simulink model "CM670A_HwAg1Meas"  (R2013b)
settings: Solver=FixedStepDiscrete  SolverMode=SingleTasking  StartTime=0.0  StopTime=22  FixedStep=0.002  RelTol=1e-3
values from neighbouring files (symbols this model uses):
  ELECGLBPRM_DEGPERREV_DEGPERREV_F32 = DataDict.Constant    [CM670A_HwAg1Meas_DataDict.m]
  ELECGLBPRM_HWAGCENTROFFS_HWDEG_F32 = DataDict.Constant    [CM670A_HwAg1Meas_DataDict.m]
  ELECGLBPRM_HWAGSATNLOWRLIM_HWDEG_F32 = DataDict.Constant    [CM670A_HwAg1Meas_DataDict.m]
  ELECGLBPRM_HWAGSATNUPPRLIM_HWDEG_F32 = DataDict.Constant    [CM670A_HwAg1Meas_DataDict.m]
  ELECGLBPRM_HWAGSCA_ULS_F32 = DataDict.Constant    [CM670A_HwAg1Meas_DataDict.m]
  ELECGLBPRM_HWAGSPURGEARRAT_ULS_F32 = DataDict.Constant    [CM670A_HwAg1Meas_DataDict.m]
  ELECGLBPRM_HWAGSPURTORINGGEARRATSNSR0_ULS_F32 = DataDict.Constant    [CM670A_HwAg1Meas_DataDict.m]
  ELECGLBPRM_HWAGSPURTORINGGEARRATSNSR1_ULS_F32 = DataDict.Constant    [CM670A_HwAg1Meas_DataDict.m]
  ELECGLBPRM_NOFLT_CNT_U08 = DataDict.Constant    [CM670A_HwAg1Meas_DataDict.m]
  ELECGLBPRM_OFFSTRIMNOTPRFMD_CNT_U08 = DataDict.Constant    [CM670A_HwAg1Meas_DataDict.m]
  ELECGLBPRM_PRTCLFLT_CNT_U08 = DataDict.Constant    [CM670A_HwAg1Meas_DataDict.m]
  ELECGLBPRM_SKIPSTEPFLT_CNT_U08 = DataDict.Constant    [CM670A_HwAg1Meas_DataDict.m]
  ELECGLBPRM_SNSRINTFLT_CNT_U08 = DataDict.Constant    [CM670A_HwAg1Meas_DataDict.m]
  ELECGLBPRM_VRNRERRFLT_CNT_U08 = DataDict.Constant    [CM670A_HwAg1Meas_DataDict.m]
  HWAG10THTOOTHTRIG_CNT_U08 = DataDict.ConfigParam    [CM670A_HwAg1Meas_DataDict.m]
  HWAG11THTOOTHTRIG_CNT_U08 = DataDict.ConfigParam    [CM670A_HwAg1Meas_DataDict.m]
  HwAg1IfFlt = DataDict.NTC    [CM670A_HwAg1Meas_DataDict.m]
  HwAg1MeasHwAg1IfFltFailStep = DataDict.Calibration    [CM670A_HwAg1Meas_DataDict.m]
  HwAg1MeasHwAg1IfFltPassStep = DataDict.Calibration    [CM670A_HwAg1Meas_DataDict.m]
  HwAg1MeasHwAg1Snsr0PrtclFltFailStep = DataDict.Calibration    [CM670A_HwAg1Meas_DataDict.m]
  HwAg1MeasHwAg1Snsr0PrtclFltPassStep = DataDict.Calibration    [CM670A_HwAg1Meas_DataDict.m]
  HwAg1MeasHwAg1Snsr1PrtclFltFailStep = DataDict.Calibration    [CM670A_HwAg1Meas_DataDict.m]
  HwAg1MeasHwAg1Snsr1PrtclFltPassStep = DataDict.Calibration    [CM670A_HwAg1Meas_DataDict.m]
  HwAg1MeasSnsr0Rev = DataDict.Calibration    [CM670A_HwAg1Meas_DataDict.m]
  HwAg1MeasSnsr1Rev = DataDict.Calibration    [CM670A_HwAg1Meas_DataDict.m]
  HwAg1MeasStep = DataDict.Calibration    [CM670A_HwAg1Meas_DataDict.m]
  HwAg1MeasVrnrErrThd = DataDict.Calibration    [CM670A_HwAg1Meas_DataDict.m]
  HwAg1MfgFlt = DataDict.NTC    [CM670A_HwAg1Meas_DataDict.m]
  HwAg1Snsr0PrtclFlt = DataDict.NTC    [CM670A_HwAg1Meas_DataDict.m]
  HwAg1Snsr1PrtclFlt = DataDict.NTC    [CM670A_HwAg1Meas_DataDict.m]
undefined symbols (not defined in the file or in its folder): NtcSts1, sigbuilder_block, SigQlfr1
libraries: simulink x30, NxtrNvM x3
(part 5 of 5)

== system CM670A_HwAg1Meas/HwAg1Meas/HwAg1MeasPer2/Snsr0Read/RawHwAgRead/NewMsg/NoStsFlt/CommFlt ==
  Action Port : ActionPort  ActionType=else
  Add : Sum
  Bus Creator1 : BusCreator  Inputs=3
  Constant : Constant  OutDataTypeStr=uint8
  CopyRight2 : Subsystem  Description=|  mask(Copyright Information){none=on}
      | Copyright info block.                                               
      |                                                                     
      | Place copyright information at the top of every subsystem in design.
      mask prompts: none "No parameters"
      mask help: Place copyright information at the top of every subsystem in design.
      mask Display:
      | NxtrConf = 'Nexteer Confidential';
      | 
      | sys = bdroot; %handle for the current model ("system")
      | first = get_param(sys,'Created');
      | first = first(end-3:end);  %year is last four digits
      | 
      | last = get_param(sys,'LastModifiedDate');
      | if isempty(last)
      |     last = datestr(now,'yyyy');
      | else
      |     last = last(end-3:end);
      | end
      | 
      | if strcmp(first,last)
      |     fprintf('%s -- Copyright %s Nexteer',NxtrConf,first)
      | else
      |     fprintf('%s -- %s%s- %s Nexteer',NxtrConf,char(169),first,last)
      | end
  Data Store Read : DataStoreRead  DataStoreName=HwAg1Snsr0IntSnsrErrCntr
  Data Store Write : DataStoreWrite  DataStoreName=HwAg1Snsr0IntSnsrErrCntr
  Data Type Conversion : DataTypeConversion  OutDataTypeStr=uint8
  Flt : Constant  Value=ELECGLBPRM_SNSRINTFLT_CNT_U08  OutDataTypeStr=uint8
  HwAg : Constant  Value=0  OutDataTypeStr=uint16
  NtcSts : simulink/Sources/Enumerated Constant  OutDataTypeStr=Enum: NtcSts1  Value=NtcSts1.NTCSTS_PREFAILD  SampleTime=inf
  Signal Conversion1 : SignalConversion
  Out2 : Outport
  wires:
  Flt/1 -> Bus Creator1/3  "ParamByte"
  NtcSts/1 -> Data Type Conversion/1
  HwAg/1 -> Bus Creator1/1  "RawHwAg"
  Bus Creator1/1 -> Signal Conversion1/1
  Signal Conversion1/1 -> Out2/1
  Data Type Conversion/1 -> Bus Creator1/2  "TestOk"
  Data Store Read/1 -> Add/1
  Constant/1 -> Add/2
  Add/1 -> Data Store Write/1

== system CM670A_HwAg1Meas/HwAg1Meas/HwAg1MeasPer2/Snsr0Read/RawHwAgRead/NewMsg/NoStsFlt/CopyRight2 ==

== system CM670A_HwAg1Meas/HwAg1Meas/HwAg1MeasPer2/Snsr0Read/RawHwAgRead/NewMsg/NoStsFlt/TestPass ==
  Snsr0Id : Inport
  Snsr0Data : Inport  Port=2
  Action Port : ActionPort  ActionType=then
  Bus Creator : BusCreator  Inputs=3
  CopyRight2 : Subsystem  Description=|  mask(Copyright Information){none=on}
      | Copyright info block.                                               
      |                                                                     
      | Place copyright information at the top of every subsystem in design.
      mask prompts: none "No parameters"
      mask help: Place copyright information at the top of every subsystem in design.
      mask Display:
      | NxtrConf = 'Nexteer Confidential';
      | 
      | sys = bdroot; %handle for the current model ("system")
      | first = get_param(sys,'Created');
      | first = first(end-3:end);  %year is last four digits
      | 
      | last = get_param(sys,'LastModifiedDate');
      | if isempty(last)
      |     last = datestr(now,'yyyy');
      | else
      |     last = last(end-3:end);
      | end
      | 
      | if strcmp(first,last)
      |     fprintf('%s -- Copyright %s Nexteer',NxtrConf,first)
      | else
      |     fprintf('%s -- %s%s- %s Nexteer',NxtrConf,char(169),first,last)
      | end
  If Action Subsystem : Subsystem  RequirementInfo={'linktype_rmi_doors' '0000cf44 (/ESG Group/FDD Module Requirements/EA4 Specific/CM670A_HwAg1Meas)' '#CM670A_49' 'true' 'REQ: CM670A_49' '' } %GIDa_aa48b249_ab70_46ce_8963_12185f434e4c  TreatAsAtomicUnit=on
  If Action Subsystem2 : Subsystem  RequirementInfo={'linktype_rmi_doors' '0000cf44 (/ESG Group/FDD Module Requirements/EA4 Specific/CM670A_HwAg1Meas)' '#CM670A_74' 'true' 'REQ: CM670A_74' '' } %GIDa_f5c78345_3720_4b83_a791_e0c886f64c70  TreatAsAtomicUnit=on
  If2 : If  IfExpression=u1 == 0
  Merge : Merge
  Merge1 : Merge
  Merge2 : Merge
  Out1 : Outport
  wires:
  Merge1/1 -> Bus Creator/2  "TestOk"
  Merge2/1 -> Bus Creator/3  "ParamByte"
  Merge/1 -> Bus Creator/1  "RawHwAg"
  Bus Creator/1 -> Out1/1
  Snsr0Id/1 -> If2/1
  If2/1 -> If Action Subsystem/Action
  If2/2 -> If Action Subsystem2/Action
  If Action Subsystem/1(RawHwAg) -> Merge/1
  If Action Subsystem2/1(RawHwAg) -> Merge/2
  If Action Subsystem/2(NtcSts) -> Merge1/1
  If Action Subsystem2/2(NtcSts) -> Merge1/2
  If Action Subsystem/3(ParamByte) -> Merge2/1
  If Action Subsystem2/3(ParamByte) -> Merge2/2
  Snsr0Data/1 -> If Action Subsystem/1(Snsr0Data)

== system CM670A_HwAg1Meas/HwAg1Meas/HwAg1MeasPer2/Snsr0Read/RawHwAgRead/NewMsg/STSFLT/CopyRight2 ==

== system CM670A_HwAg1Meas/HwAg1Meas/HwAg1MeasPer3/Snsr1Read/RawHwAgRead/NewMsg/NoStsFlt/CommFlt ==
  Action Port : ActionPort  ActionType=else
  Add : Sum
  Bus Creator1 : BusCreator  Inputs=3
  Constant : Constant  OutDataTypeStr=uint8
  CopyRight2 : Subsystem  Description=|  mask(Copyright Information){none=on}
      | Copyright info block.                                               
      |                                                                     
      | Place copyright information at the top of every subsystem in design.
      mask prompts: none "No parameters"
      mask help: Place copyright information at the top of every subsystem in design.
      mask Display:
      | NxtrConf = 'Nexteer Confidential';
      | 
      | sys = bdroot; %handle for the current model ("system")
      | first = get_param(sys,'Created');
      | first = first(end-3:end);  %year is last four digits
      | 
      | last = get_param(sys,'LastModifiedDate');
      | if isempty(last)
      |     last = datestr(now,'yyyy');
      | else
      |     last = last(end-3:end);
      | end
      | 
      | if strcmp(first,last)
      |     fprintf('%s -- Copyright %s Nexteer',NxtrConf,first)
      | else
      |     fprintf('%s -- %s%s- %s Nexteer',NxtrConf,char(169),first,last)
      | end
  Data Store Read : DataStoreRead  DataStoreName=HwAg1Snsr1IntSnsrErrCntr
  Data Store Write : DataStoreWrite  DataStoreName=HwAg1Snsr1IntSnsrErrCntr
  Data Type Conversion : DataTypeConversion  OutDataTypeStr=uint8
  Flt : Constant  Value=ELECGLBPRM_SNSRINTFLT_CNT_U08  OutDataTypeStr=uint8
  HwAg : Constant  Value=0  OutDataTypeStr=uint16
  NtcSts : simulink/Sources/Enumerated Constant  OutDataTypeStr=Enum: NtcSts1  Value=NtcSts1.NTCSTS_PREFAILD  SampleTime=inf
  Signal Conversion1 : SignalConversion
  Out2 : Outport
  wires:
  Flt/1 -> Bus Creator1/3  "ParamByte"
  NtcSts/1 -> Data Type Conversion/1
  HwAg/1 -> Bus Creator1/1  "RawHwAg"
  Bus Creator1/1 -> Signal Conversion1/1
  Signal Conversion1/1 -> Out2/1
  Data Type Conversion/1 -> Bus Creator1/2  "TestOk"
  Data Store Read/1 -> Add/1
  Constant/1 -> Add/2
  Add/1 -> Data Store Write/1

== system CM670A_HwAg1Meas/HwAg1Meas/HwAg1MeasPer3/Snsr1Read/RawHwAgRead/NewMsg/NoStsFlt/CopyRight2 ==

== system CM670A_HwAg1Meas/HwAg1Meas/HwAg1MeasPer3/Snsr1Read/RawHwAgRead/NewMsg/NoStsFlt/TestPass ==
  Snsr1Id : Inport
  Snsr1Data : Inport  Port=2
  Action Port : ActionPort  ActionType=then
  Bus Creator : BusCreator  Inputs=3
  CopyRight2 : Subsystem  Description=|  mask(Copyright Information){none=on}
      | Copyright info block.                                               
      |                                                                     
      | Place copyright information at the top of every subsystem in design.
      mask prompts: none "No parameters"
      mask help: Place copyright information at the top of every subsystem in design.
      mask Display:
      | NxtrConf = 'Nexteer Confidential';
      | 
      | sys = bdroot; %handle for the current model ("system")
      | first = get_param(sys,'Created');
      | first = first(end-3:end);  %year is last four digits
      | 
      | last = get_param(sys,'LastModifiedDate');
      | if isempty(last)
      |     last = datestr(now,'yyyy');
      | else
      |     last = last(end-3:end);
      | end
      | 
      | if strcmp(first,last)
      |     fprintf('%s -- Copyright %s Nexteer',NxtrConf,first)
      | else
      |     fprintf('%s -- %s%s- %s Nexteer',NxtrConf,char(169),first,last)
      | end
  If Action Subsystem : Subsystem  RequirementInfo={'linktype_rmi_doors' '0000cf44 (/ESG Group/FDD Module Requirements/EA4 Specific/CM670A_HwAg1Meas)' '#CM670A_73' 'true' 'REQ: CM670A_73' '' } %GIDa_606bd5a3_5e49_4a65_919f_9ded041dacb2  TreatAsAtomicUnit=on
  If Action Subsystem2 : Subsystem  RequirementInfo={'linktype_rmi_doors' '0000cf44 (/ESG Group/FDD Module Requirements/EA4 Specific/CM670A_HwAg1Meas)' '#CM670A_75' 'true' 'REQ: CM670A_75' '' } %GIDa_005b1b66_d003_4573_abd6_345df925bde0  TreatAsAtomicUnit=on
  If2 : If  IfExpression=u1 == 1
  Merge : Merge
  Merge1 : Merge
  Merge2 : Merge
  Out1 : Outport
  wires:
  Merge1/1 -> Bus Creator/2  "TestOk"
  Merge2/1 -> Bus Creator/3  "ParamByte"
  Merge/1 -> Bus Creator/1  "RawHwAg"
  Bus Creator/1 -> Out1/1
  Snsr1Id/1 -> If2/1
  If2/1 -> If Action Subsystem/Action
  If2/2 -> If Action Subsystem2/Action
  If Action Subsystem/1(RawHwAg) -> Merge/1
  If Action Subsystem2/1(RawHwAg) -> Merge/2
  If Action Subsystem/2(NtcSts) -> Merge1/1
  If Action Subsystem2/2(NtcSts) -> Merge1/2
  If Action Subsystem/3(ParamByte) -> Merge2/1
  If Action Subsystem2/3(ParamByte) -> Merge2/2
  Snsr1Data/1 -> If Action Subsystem/1(Snsr1Data)

== system CM670A_HwAg1Meas/HwAg1Meas/HwAg1MeasPer3/Snsr1Read/RawHwAgRead/NewMsg/STSFLT/CopyRight2 ==

== system CM670A_HwAg1Meas/HwAg1Meas/HwAg1MeasPer4/HwAgRead/If Action Subsystem/AdjStepCalc/Diagc/CopyRight2 ==

== system CM670A_HwAg1Meas/HwAg1Meas/HwAg1MeasPer4/HwAgRead/If Action Subsystem/AdjStepCalc/Diagc/If Action  ==
  HwAg1Snsr0Rev : Inport
  HwAg1Snsr1Rev : Inport  Port=2
  HwAg1Snsr0Rel : Inport  Port=3
  HwAg1Snsr1Rel : Inport  Port=4
  HwAg1StepSeqNr : Inport  Port=5
  Action Port : ActionPort  ActionType=then
  AbsCalcHwAg1Snsr0 : Subsystem
  AbsCalcHwAg1Snsr1 : Subsystem
  CopyRight2 : Subsystem  Description=|  mask(Copyright Information){none=on}
      | Copyright info block.                                               
      |                                                                     
      | Place copyright information at the top of every subsystem in design.
      mask prompts: none "No parameters"
      mask help: Place copyright information at the top of every subsystem in design.
      mask Display:
      | NxtrConf = 'Nexteer Confidential';
      | 
      | sys = bdroot; %handle for the current model ("system")
      | first = get_param(sys,'Created');
      | first = first(end-3:end);  %year is last four digits
      | 
      | last = get_param(sys,'LastModifiedDate');
      | if isempty(last)
      |     last = datestr(now,'yyyy');
      | else
      |     last = last(end-3:end);
      | end
      | 
      | if strcmp(first,last)
      |     fprintf('%s -- Copyright %s Nexteer',NxtrConf,first)
      | else
      |     fprintf('%s -- %s%s- %s Nexteer',NxtrConf,char(169),first,last)
      | end
  PIM : DataStoreWrite  DataStoreName=HwAg1PrevStepSeqNr
  finalAbsAg : Subsystem
  HwAg1Meas : Outport
  HwAg1TestOk : Outport  Port=2
  ParamByte : Outport  Port=3
  wires:
  HwAg1Snsr0Rev/1 -> AbsCalcHwAg1Snsr0/2(HwAg1Snsr0Rev)
  AbsCalcHwAg1Snsr0/1(HwAg1Snsr0Abs) -> finalAbsAg/1(HwAg1Snsr0Abs)
  AbsCalcHwAg1Snsr1/1(HwAg1Snsr1Abs) -> finalAbsAg/2(HwAg1Snsr1Abs)
  finalAbsAg/1(HwAg1) -> HwAg1Meas/1
  finalAbsAg/2(TestOk) -> HwAg1TestOk/1
  finalAbsAg/3(ParamByte) -> ParamByte/1
  HwAg1Snsr0Rel/1 -> AbsCalcHwAg1Snsr0/1(HwAg1Snsr0Rel)
  HwAg1StepSeqNr/1 -> PIM/1
  HwAg1Snsr1Rel/1 -> AbsCalcHwAg1Snsr1/1(HwAg1Snsr1Rel)
  HwAg1Snsr1Rev/1 -> AbsCalcHwAg1Snsr1/2(HwAg1Snsr1Rev)

== system CM670A_HwAg1Meas/HwAg1Meas/HwAg1MeasPer4/HwAgRead/If Action Subsystem/AdjStepCalc/Diagc/If Action Skip ==
  Action Port : ActionPort  ActionType=else
  CopyRight2 : Subsystem  Description=|  mask(Copyright Information){none=on}
      | Copyright info block.                                               
      |                                                                     
      | Place copyright information at the top of every subsystem in design.
      mask prompts: none "No parameters"
      mask help: Place copyright information at the top of every subsystem in design.
      mask Display:
      | NxtrConf = 'Nexteer Confidential';
      | 
      | sys = bdroot; %handle for the current model ("system")
      | first = get_param(sys,'Created');
      | first = first(end-3:end);  %year is last four digits
      | 
      | last = get_param(sys,'LastModifiedDate');
      | if isempty(last)
      |     last = datestr(now,'yyyy');
      | else
      |     last = last(end-3:end);
      | end
      | 
      | if strcmp(first,last)
      |     fprintf('%s -- Copyright %s Nexteer',NxtrConf,first)
      | else
      |     fprintf('%s -- %s%s- %s Nexteer',NxtrConf,char(169),first,last)
      | end
  Data Type Conversion : DataTypeConversion  OutDataTypeStr=uint8
  Flt : Constant  Value=ELECGLBPRM_SKIPSTEPFLT_CNT_U08  OutDataTypeStr=uint8
  HwAg1 : Constant  Value=0  OutDataTypeStr=single
  NtcSts : simulink/Sources/Enumerated Constant  OutDataTypeStr=Enum: NtcSts1  Value=NtcSts1.NTCSTS_PREFAILD  SampleTime=inf
  HwAg1Meas : Outport
  HwAg1TestOk : Outport  Port=2  OutDataTypeStr=uint8
  ParamByte : Outport  Port=3
  wires:
  NtcSts/1 -> Data Type Conversion/1
  Flt/1 -> ParamByte/1
  HwAg1/1 -> HwAg1Meas/1
  Data Type Conversion/1 -> HwAg1TestOk/1

== system CM670A_HwAg1Meas/HwAg1Meas/HwAg1MeasPer4/HwAgRead/If Action Subsystem/AdjStepCalc/InitStep/CopyRight2 ==

== system CM670A_HwAg1Meas/HwAg1Meas/HwAg1MeasPer4/HwAgRead/If Action Subsystem/AdjStepCalc/InitStep/DoNothing ==
  Action Port : ActionPort  ActionType=else
  CopyRight2 : Subsystem  Description=|  mask(Copyright Information){none=on}
      | Copyright info block.                                               
      |                                                                     
      | Place copyright information at the top of every subsystem in design.
      mask prompts: none "No parameters"
      mask help: Place copyright information at the top of every subsystem in design.
      mask Display:
      | NxtrConf = 'Nexteer Confidential';
      | 
      | sys = bdroot; %handle for the current model ("system")
      | first = get_param(sys,'Created');
      | first = first(end-3:end);  %year is last four digits
      | 
      | last = get_param(sys,'LastModifiedDate');
      | if isempty(last)
      |     last = datestr(now,'yyyy');
      | else
      |     last = last(end-3:end);
      | end
      | 
      | if strcmp(first,last)
      |     fprintf('%s -- Copyright %s Nexteer',NxtrConf,first)
      | else
      |     fprintf('%s -- %s%s- %s Nexteer',NxtrConf,char(169),first,last)
      | end

== system CM670A_HwAg1Meas/HwAg1Meas/HwAg1MeasPer4/HwAgRead/If Action Subsystem/AdjStepCalc/InitStep/Else ==
  HwAg1StepSeqNr : Inport
  Action Port : ActionPort  ActionType=then
  Constant : Constant  OutDataTypeStr=boolean
  CopyRight2 : Subsystem  Description=|  mask(Copyright Information){none=on}
      | Copyright info block.                                               
      |                                                                     
      | Place copyright information at the top of every subsystem in design.
      mask prompts: none "No parameters"
      mask help: Place copyright information at the top of every subsystem in design.
      mask Display:
      | NxtrConf = 'Nexteer Confidential';
      | 
      | sys = bdroot; %handle for the current model ("system")
      | first = get_param(sys,'Created');
      | first = first(end-3:end);  %year is last four digits
      | 
      | last = get_param(sys,'LastModifiedDate');
      | if isempty(last)
      |     last = datestr(now,'yyyy');
      | else
      |     last = last(end-3:end);
      | end
      | 
      | if strcmp(first,last)
      |     fprintf('%s -- Copyright %s Nexteer',NxtrConf,first)
      | else
      |     fprintf('%s -- %s%s- %s Nexteer',NxtrConf,char(169),first,last)
      | end
  PIM : DataStoreWrite  DataStoreName=HwAg1PrevStepSeqNr
  PIM1 : DataStoreWrite  DataStoreName=HwAg1InitStepSeqNrCmpl
  wires:
  HwAg1StepSeqNr/1 -> PIM/1
  Constant/1 -> PIM1/1

== system CM670A_HwAg1Meas/HwAg1Meas/HwAg1MeasPer4/HwAgRead/If Action Subsystem/AdjStepCalc/Intpn/CopyRight2 ==

== system CM670A_HwAg1Meas/HwAg1Meas/HwAg1MeasPer4/HwAgRead/If Action Subsystem/AdjStepCalc/Intpn/StepCalc ==
  HwAg1Snsr0Rel : Inport
  HwAg1Snsr1Rel : Inport  Port=2
  Add : Sum  Inputs=+-
  CopyRight2 : Subsystem  Description=|  mask(Copyright Information){none=on}
      | Copyright info block.                                               
      |                                                                     
      | Place copyright information at the top of every subsystem in design.
      mask prompts: none "No parameters"
      mask help: Place copyright information at the top of every subsystem in design.
      mask Display:
      | NxtrConf = 'Nexteer Confidential';
      | 
      | sys = bdroot; %handle for the current model ("system")
      | first = get_param(sys,'Created');
      | first = first(end-3:end);  %year is last four digits
      | 
      | last = get_param(sys,'LastModifiedDate');
      | if isempty(last)
      |     last = datestr(now,'yyyy');
      | else
      |     last = last(end-3:end);
      | end
      | 
      | if strcmp(first,last)
      |     fprintf('%s -- Copyright %s Nexteer',NxtrConf,first)
      | else
      |     fprintf('%s -- %s%s- %s Nexteer',NxtrConf,char(169),first,last)
      | end
  Data Type Conversion1 : DataTypeConversion  OutDataTypeStr=single
  HwAgSpurGearRat : Constant  Value=ELECGLBPRM_HWAGSPURGEARRAT_ULS_F32  OutDataTypeStr=single
  Product : Product
  Scope : Scope  NumInputPorts=4
      settings: ShowLegends=on  TimeRange=10  YMin=0~0~0~-150  YMax=400~400~400~350  SaveName=ScopeData10
  HwAg1Step : Outport  OutDataTypeStr=single
  wires:
  Data Type Conversion1/1 -> Product/1
  Product/1 -> Add/2, Scope/3  "Snsr1Multi"
  HwAgSpurGearRat/1 -> Product/2
  Add/1 -> Scope/4, HwAg1Step/1  "StepVal"
  HwAg1Snsr1Rel/1 -> Data Type Conversion1/1, Scope/2  "Snsr1Rel"
  HwAg1Snsr0Rel/1 -> Scope/1, Add/1  "Snsr0Rel"

== system CM670A_HwAg1Meas/HwAg1Meas/HwAg1MeasPer2/Snsr0Read/RawHwAgRead/NewMsg/NoStsFlt/CommFlt/CopyRight2 ==

== system CM670A_HwAg1Meas/HwAg1Meas/HwAg1MeasPer2/Snsr0Read/RawHwAgRead/NewMsg/NoStsFlt/TestPass/CopyRight2 ==

== system CM670A_HwAg1Meas/HwAg1Meas/HwAg1MeasPer2/Snsr0Read/RawHwAgRead/NewMsg/NoStsFlt/TestPass/If Action Subsystem ==
  note: Information only:
      |
      | - Correct Sensor As identified
  Snsr0Data : Inport
  Action Port : ActionPort  ActionType=then
  CopyRight2 : Subsystem  Description=|  mask(Copyright Information){none=on}
      | Copyright info block.                                               
      |                                                                     
      | Place copyright information at the top of every subsystem in design.
      mask prompts: none "No parameters"
      mask help: Place copyright information at the top of every subsystem in design.
      mask Display:
      | NxtrConf = 'Nexteer Confidential';
      | 
      | sys = bdroot; %handle for the current model ("system")
      | first = get_param(sys,'Created');
      | first = first(end-3:end);  %year is last four digits
      | 
      | last = get_param(sys,'LastModifiedDate');
      | if isempty(last)
      |     last = datestr(now,'yyyy');
      | else
      |     last = last(end-3:end);
      | end
      | 
      | if strcmp(first,last)
      |     fprintf('%s -- Copyright %s Nexteer',NxtrConf,first)
      | else
      |     fprintf('%s -- %s%s- %s Nexteer',NxtrConf,char(169),first,last)
      | end
  Data Type Conversion : DataTypeConversion  OutDataTypeStr=uint8
  NoFlt : Constant  RequirementInfo={} %GIDa_fc544854_ed19_421f_ad77_015280455b5f  Value=ELECGLBPRM_NOFLT_CNT_U08  OutDataTypeStr=uint8
  NtcSts1 : simulink/Sources/Enumerated Constant  OutDataTypeStr=Enum: NtcSts1  Value=NtcSts1.NTCSTS_PREPASSD  SampleTime=inf
  RawHwAg : Outport
  NtcSts : Outport  Port=2
  ParamByte : Outport  Port=3
  wires:
  NtcSts1/1 -> Data Type Conversion/1
  Snsr0Data/1 -> RawHwAg/1
  NoFlt/1 -> ParamByte/1
  Data Type Conversion/1 -> NtcSts/1

== system CM670A_HwAg1Meas/HwAg1Meas/HwAg1MeasPer2/Snsr0Read/RawHwAgRead/NewMsg/NoStsFlt/TestPass/If Action Subsystem2 ==
  note: Information only:
      |
      | - Perform Diagnostic If not expected, Sensor is out of Sync
  Action Port : ActionPort  ActionType=else
  Add : Sum
  Constant : Constant  OutDataTypeStr=uint8
  CopyRight2 : Subsystem  Description=|  mask(Copyright Information){none=on}
      | Copyright info block.                                               
      |                                                                     
      | Place copyright information at the top of every subsystem in design.
      mask prompts: none "No parameters"
      mask help: Place copyright information at the top of every subsystem in design.
      mask Display:
      | NxtrConf = 'Nexteer Confidential';
      | 
      | sys = bdroot; %handle for the current model ("system")
      | first = get_param(sys,'Created');
      | first = first(end-3:end);  %year is last four digits
      | 
      | last = get_param(sys,'LastModifiedDate');
      | if isempty(last)
      |     last = datestr(now,'yyyy');
      | else
      |     last = last(end-3:end);
      | end
      | 
      | if strcmp(first,last)
      |     fprintf('%s -- Copyright %s Nexteer',NxtrConf,first)
      | else
      |     fprintf('%s -- %s%s- %s Nexteer',NxtrConf,char(169),first,last)
      | end
  Data Store Read : DataStoreRead  DataStoreName=HwAg1Snsr0IdErrCntr
  Data Store Write : DataStoreWrite  DataStoreName=HwAg1Snsr0IdErrCntr
  Data Type Conversion : DataTypeConversion  OutDataTypeStr=uint8
  HwAg : Constant  Value=0  OutDataTypeStr=uint16
  NtcSts1 : simulink/Sources/Enumerated Constant  OutDataTypeStr=Enum: NtcSts1  Value=NtcSts1.NTCSTS_PREFAILD  SampleTime=inf
  PRTCL_FAULT : Constant  Value=ELECGLBPRM_PRTCLFLT_CNT_U08  OutDataTypeStr=uint8
  RawHwAg : Outport
  NtcSts : Outport  Port=2
  ParamByte : Outport  Port=3
  wires:
  HwAg/1 -> RawHwAg/1
  NtcSts1/1 -> Data Type Conversion/1
  PRTCL_FAULT/1 -> ParamByte/1
  Data Type Conversion/1 -> NtcSts/1
  Data Store Read/1 -> Add/1
  Constant/1 -> Add/2
  Add/1 -> Data Store Write/1

== system CM670A_HwAg1Meas/HwAg1Meas/HwAg1MeasPer3/Snsr1Read/RawHwAgRead/NewMsg/NoStsFlt/CommFlt/CopyRight2 ==

== system CM670A_HwAg1Meas/HwAg1Meas/HwAg1MeasPer3/Snsr1Read/RawHwAgRead/NewMsg/NoStsFlt/TestPass/CopyRight2 ==

== system CM670A_HwAg1Meas/HwAg1Meas/HwAg1MeasPer3/Snsr1Read/RawHwAgRead/NewMsg/NoStsFlt/TestPass/If Action Subsystem ==
  note: Information only:
      |
      | - Correct Sensor As identified
  Snsr1Data : Inport
  Action Port : ActionPort  ActionType=then
  CopyRight2 : Subsystem  Description=|  mask(Copyright Information){none=on}
      | Copyright info block.                                               
      |                                                                     
      | Place copyright information at the top of every subsystem in design.
      mask prompts: none "No parameters"
      mask help: Place copyright information at the top of every subsystem in design.
      mask Display:
      | NxtrConf = 'Nexteer Confidential';
      | 
      | sys = bdroot; %handle for the current model ("system")
      | first = get_param(sys,'Created');
      | first = first(end-3:end);  %year is last four digits
      | 
      | last = get_param(sys,'LastModifiedDate');
      | if isempty(last)
      |     last = datestr(now,'yyyy');
      | else
      |     last = last(end-3:end);
      | end
      | 
      | if strcmp(first,last)
      |     fprintf('%s -- Copyright %s Nexteer',NxtrConf,first)
      | else
      |     fprintf('%s -- %s%s- %s Nexteer',NxtrConf,char(169),first,last)
      | end
  Data Type Conversion : DataTypeConversion  OutDataTypeStr=uint8
  NoFlt : Constant  RequirementInfo={} %GIDa_d748ad04_0454_4909_8f3a_7760530ce8d7  Value=ELECGLBPRM_NOFLT_CNT_U08  OutDataTypeStr=uint8
  NtcSts1 : simulink/Sources/Enumerated Constant  OutDataTypeStr=Enum: NtcSts1  Value=NtcSts1.NTCSTS_PREPASSD  SampleTime=inf
  RawHwAg : Outport
  NtcSts : Outport  Port=2
  ParamByte : Outport  Port=3
  wires:
  NtcSts1/1 -> Data Type Conversion/1
  Snsr1Data/1 -> RawHwAg/1
  NoFlt/1 -> ParamByte/1
  Data Type Conversion/1 -> NtcSts/1

== system CM670A_HwAg1Meas/HwAg1Meas/HwAg1MeasPer3/Snsr1Read/RawHwAgRead/NewMsg/NoStsFlt/TestPass/If Action Subsystem2 ==
  note: Information Purpose Only :
      |
      | Sensor Sending Message Out of Order or 11th Tooth Sensor not Responding
  Action Port : ActionPort  ActionType=else
  Add : Sum
  Constant : Constant  OutDataTypeStr=uint8
  CopyRight2 : Subsystem  Description=|  mask(Copyright Information){none=on}
      | Copyright info block.                                               
      |                                                                     
      | Place copyright information at the top of every subsystem in design.
      mask prompts: none "No parameters"
      mask help: Place copyright information at the top of every subsystem in design.
      mask Display:
      | NxtrConf = 'Nexteer Confidential';
      | 
      | sys = bdroot; %handle for the current model ("system")
      | first = get_param(sys,'Created');
      | first = first(end-3:end);  %year is last four digits
      | 
      | last = get_param(sys,'LastModifiedDate');
      | if isempty(last)
      |     last = datestr(now,'yyyy');
      | else
      |     last = last(end-3:end);
      | end
      | 
      | if strcmp(first,last)
      |     fprintf('%s -- Copyright %s Nexteer',NxtrConf,first)
      | else
      |     fprintf('%s -- %s%s- %s Nexteer',NxtrConf,char(169),first,last)
      | end
  Data Store Read : DataStoreRead  DataStoreName=HwAg1Snsr1IdErrCntr
  Data Store Write : DataStoreWrite  DataStoreName=HwAg1Snsr1IdErrCntr
  Data Type Conversion : DataTypeConversion  OutDataTypeStr=uint8
  HwAg : Constant  Value=0  OutDataTypeStr=uint16
  NtcSts1 : simulink/Sources/Enumerated Constant  OutDataTypeStr=Enum: NtcSts1  Value=NtcSts1.NTCSTS_PREFAILD  SampleTime=inf
  PRTCL_FAULT : Constant  Value=ELECGLBPRM_PRTCLFLT_CNT_U08  OutDataTypeStr=uint8
  RawHwAg : Outport
  NtcSts : Outport  Port=2
  ParamByte : Outport  Port=3
  wires:
  HwAg/1 -> RawHwAg/1
  NtcSts1/1 -> Data Type Conversion/1
  PRTCL_FAULT/1 -> ParamByte/1
  Data Type Conversion/1 -> NtcSts/1
  Data Store Read/1 -> Add/1
  Constant/1 -> Add/2
  Add/1 -> Data Store Write/1

== system CM670A_HwAg1Meas/HwAg1Meas/HwAg1MeasPer4/HwAgRead/If Action Subsystem/AdjStepCalc/Diagc/If Action /AbsCalcHwAg1Snsr0 ==
  HwAg1Snsr0Rel : Inport
  HwAg1Snsr0Rev : Inport  Port=2
  Add : Sum
  CopyRight2 : Subsystem  Description=|  mask(Copyright Information){none=on}
      | Copyright info block.                                               
      |                                                                     
      | Place copyright information at the top of every subsystem in design.
      mask prompts: none "No parameters"
      mask help: Place copyright information at the top of every subsystem in design.
      mask Display:
      | NxtrConf = 'Nexteer Confidential';
      | 
      | sys = bdroot; %handle for the current model ("system")
      | first = get_param(sys,'Created');
      | first = first(end-3:end);  %year is last four digits
      | 
      | last = get_param(sys,'LastModifiedDate');
      | if isempty(last)
      |     last = datestr(now,'yyyy');
      | else
      |     last = last(end-3:end);
      | end
      | 
      | if strcmp(first,last)
      |     fprintf('%s -- Copyright %s Nexteer',NxtrConf,first)
      | else
      |     fprintf('%s -- %s%s- %s Nexteer',NxtrConf,char(169),first,last)
      | end
  HwAgRevDeg : Constant  Value=ELECGLBPRM_DEGPERREV_DEGPERREV_F32  OutDataTypeStr=single
  HwAgRevDeg2 : Constant  Value=ELECGLBPRM_HWAGSPURTORINGGEARRATSNSR0_ULS_F32  OutDataTypeStr=single
  PIM : DataStoreWrite  RequirementInfo={} %GIDa_f9686ddf_6d7f_4bd7_aab0_69657c52dad4  DataStoreName=dHwAg1MeasSnsr0Abs
  Product : Product
  Product1 : Product
  HwAg1Snsr0Abs : Outport  OutDataTypeStr=single
  wires:
  HwAg1Snsr0Rev/1 -> Product/1
  HwAgRevDeg/1 -> Product/2
  HwAg1Snsr0Rel/1 -> Add/1
  Product/1 -> Add/2
  Add/1 -> Product1/1
  Product1/1 -> PIM/1, HwAg1Snsr0Abs/1
  HwAgRevDeg2/1 -> Product1/2

== system CM670A_HwAg1Meas/HwAg1Meas/HwAg1MeasPer4/HwAgRead/If Action Subsystem/AdjStepCalc/Diagc/If Action /AbsCalcHwAg1Snsr1 ==
  HwAg1Snsr1Rel : Inport
  HwAg1Snsr1Rev : Inport  Port=2
  Add : Sum
  CopyRight2 : Subsystem  Description=|  mask(Copyright Information){none=on}
      | Copyright info block.                                               
      |                                                                     
      | Place copyright information at the top of every subsystem in design.
      mask prompts: none "No parameters"
      mask help: Place copyright information at the top of every subsystem in design.
      mask Display:
      | NxtrConf = 'Nexteer Confidential';
      | 
      | sys = bdroot; %handle for the current model ("system")
      | first = get_param(sys,'Created');
      | first = first(end-3:end);  %year is last four digits
      | 
      | last = get_param(sys,'LastModifiedDate');
      | if isempty(last)
      |     last = datestr(now,'yyyy');
      | else
      |     last = last(end-3:end);
      | end
      | 
      | if strcmp(first,last)
      |     fprintf('%s -- Copyright %s Nexteer',NxtrConf,first)
      | else
      |     fprintf('%s -- %s%s- %s Nexteer',NxtrConf,char(169),first,last)
      | end
  HwAgRevDeg : Constant  Value=ELECGLBPRM_DEGPERREV_DEGPERREV_F32  OutDataTypeStr=single
  HwAgRevDeg1 : Constant  Value=ELECGLBPRM_HWAGSPURTORINGGEARRATSNSR1_ULS_F32  OutDataTypeStr=single
  PIM : DataStoreWrite  RequirementInfo={} %GIDa_948d4c45_9707_430a_97e1_17fee5f64561  DataStoreName=dHwAg1MeasSnsr1Abs
  Product : Product
  Product1 : Product
  HwAg1Snsr1Abs : Outport  OutDataTypeStr=single
  wires:
  HwAg1Snsr1Rev/1 -> Product/1
  HwAgRevDeg/1 -> Product/2
  HwAg1Snsr1Rel/1 -> Add/1
  Product/1 -> Add/2
  Add/1 -> Product1/1
  HwAgRevDeg1/1 -> Product1/2
  Product1/1 -> PIM/1, HwAg1Snsr1Abs/1

== system CM670A_HwAg1Meas/HwAg1Meas/HwAg1MeasPer4/HwAgRead/If Action Subsystem/AdjStepCalc/Diagc/If Action /CopyRight2 ==

== system CM670A_HwAg1Meas/HwAg1Meas/HwAg1MeasPer4/HwAgRead/If Action Subsystem/AdjStepCalc/Diagc/If Action /finalAbsAg ==
  HwAg1Snsr0Abs : Inport
  HwAg1Snsr1Abs : Inport  Port=2
  Abs : Abs
  Constant1 : Constant  Value=HwAg1MeasVrnrErrThd
  CopyRight2 : Subsystem  Description=|  mask(Copyright Information){none=on}
      | Copyright info block.                                               
      |                                                                     
      | Place copyright information at the top of every subsystem in design.
      mask prompts: none "No parameters"
      mask help: Place copyright information at the top of every subsystem in design.
      mask Display:
      | NxtrConf = 'Nexteer Confidential';
      | 
      | sys = bdroot; %handle for the current model ("system")
      | first = get_param(sys,'Created');
      | first = first(end-3:end);  %year is last four digits
      | 
      | last = get_param(sys,'LastModifiedDate');
      | if isempty(last)
      |     last = datestr(now,'yyyy');
      | else
      |     last = last(end-3:end);
      | end
      | 
      | if strcmp(first,last)
      |     fprintf('%s -- Copyright %s Nexteer',NxtrConf,first)
      | else
      |     fprintf('%s -- %s%s- %s Nexteer',NxtrConf,char(169),first,last)
      | end
  Data Type Conversion : DataTypeConversion  OutDataTypeStr=single
  If : If  NumInputs=2  IfExpression=u1 < u2
  If Action Subsystem : Subsystem  RequirementInfo={'linktype_rmi_doors' '0000cf44 (/ESG Group/FDD Module Requirements/EA4 Specific/CM670A_HwAg1Meas)' '#CM670A_100' 'true' 'REQ: CM670A_100' '' } %GIDa_5cb80530_28a1_4b53_9327_5ab76c29c726  TreatAsAtomicUnit=on
  If Action Subsystem1 : Subsystem  RequirementInfo={'linktype_rmi_doors' '0000cf44 (/ESG Group/FDD Module Requirements/EA4 Specific/CM670A_HwAg1Meas)' '#CM670A_98' 'true' 'REQ: CM670A_98' '' } %GIDa_4afdd560_1f19_433e_8fad_f8f509705c15  TreatAsAtomicUnit=on
  Merge : Merge
  Merge1 : Merge
  Merge2 : Merge
  Scope : Scope  NumInputPorts=3
      settings: TimeRange=10  YMin=100~0~0  YMax=750~65000~65000  SaveName=ScopeData7
  Sub : Sum  Inputs=+-
  HwAg1 : Outport  OutDataTypeStr=single
  TestOk : Outport  Port=2  OutDataTypeStr=uint8
  ParamByte : Outport  Port=3  OutDataTypeStr=uint8
  wires:
  HwAg1Snsr0Abs/1 -> Scope/1, If Action Subsystem/1(HwAg1Snsr0Abs), Sub/1  "Snsr0Abs"
  HwAg1Snsr1Abs/1 -> Scope/2, If Action Subsystem/2(HwAg1Snsr1Abs), Sub/2  "Snsr1Abs"
  Sub/1 -> Abs/1
  Abs/1 -> Scope/3, If/1  "VernierAbs"
  Constant1/1 -> Data Type Conversion/1
  If/1 -> If Action Subsystem/Action
  If/2 -> If Action Subsystem1/Action
  If Action Subsystem1/2(HwAg1TestOk) -> Merge/2
  If Action Subsystem/2(HwAg1TestOk) -> Merge/1
  Merge/1 -> TestOk/1
  If Action Subsystem/1(HwAg1Meas) -> Merge1/1
  If Action Subsystem/3(ParamByte) -> Merge2/1
  If Action Subsystem1/1(HwAg1Meas) -> Merge1/2
  If Action Subsystem1/3(ParamByte) -> Merge2/2
  Merge2/1 -> ParamByte/1
  Merge1/1 -> HwAg1/1
  Data Type Conversion/1 -> If/2

== system CM670A_HwAg1Meas/HwAg1Meas/HwAg1MeasPer4/HwAgRead/If Action Subsystem/AdjStepCalc/Diagc/If Action Skip/CopyRight2 ==

== system CM670A_HwAg1Meas/HwAg1Meas/HwAg1MeasPer4/HwAgRead/If Action Subsystem/AdjStepCalc/InitStep/DoNothing/CopyRight2 ==

== system CM670A_HwAg1Meas/HwAg1Meas/HwAg1MeasPer4/HwAgRead/If Action Subsystem/AdjStepCalc/InitStep/Else/CopyRight2 ==

== system CM670A_HwAg1Meas/HwAg1Meas/HwAg1MeasPer4/HwAgRead/If Action Subsystem/AdjStepCalc/Intpn/StepCalc/CopyRight2 ==

== system CM670A_HwAg1Meas/HwAg1Meas/HwAg1MeasPer2/Snsr0Read/RawHwAgRead/NewMsg/NoStsFlt/TestPass/If Action Subsystem/CopyRight2 ==

== system CM670A_HwAg1Meas/HwAg1Meas/HwAg1MeasPer2/Snsr0Read/RawHwAgRead/NewMsg/NoStsFlt/TestPass/If Action Subsystem2/CopyRight2 ==

== system CM670A_HwAg1Meas/HwAg1Meas/HwAg1MeasPer3/Snsr1Read/RawHwAgRead/NewMsg/NoStsFlt/TestPass/If Action Subsystem/CopyRight2 ==

== system CM670A_HwAg1Meas/HwAg1Meas/HwAg1MeasPer3/Snsr1Read/RawHwAgRead/NewMsg/NoStsFlt/TestPass/If Action Subsystem2/CopyRight2 ==

== system CM670A_HwAg1Meas/HwAg1Meas/HwAg1MeasPer4/HwAgRead/If Action Subsystem/AdjStepCalc/Diagc/If Action /AbsCalcHwAg1Snsr0/CopyRight2 ==

== system CM670A_HwAg1Meas/HwAg1Meas/HwAg1MeasPer4/HwAgRead/If Action Subsystem/AdjStepCalc/Diagc/If Action /AbsCalcHwAg1Snsr1/CopyRight2 ==

== system CM670A_HwAg1Meas/HwAg1Meas/HwAg1MeasPer4/HwAgRead/If Action Subsystem/AdjStepCalc/Diagc/If Action /finalAbsAg/CopyRight2 ==

== system CM670A_HwAg1Meas/HwAg1Meas/HwAg1MeasPer4/HwAgRead/If Action Subsystem/AdjStepCalc/Diagc/If Action /finalAbsAg/If Action Subsystem ==
  HwAg1Snsr0Abs : Inport
  HwAg1Snsr1Abs : Inport  Port=2
  Action Port : ActionPort  ActionType=then
  Add : Sum
  Add1 : Sum  Inputs=+-
  CopyRight2 : Subsystem  Description=|  mask(Copyright Information){none=on}
      | Copyright info block.                                               
      |                                                                     
      | Place copyright information at the top of every subsystem in design.
      mask prompts: none "No parameters"
      mask help: Place copyright information at the top of every subsystem in design.
      mask Display:
      | NxtrConf = 'Nexteer Confidential';
      | 
      | sys = bdroot; %handle for the current model ("system")
      | first = get_param(sys,'Created');
      | first = first(end-3:end);  %year is last four digits
      | 
      | last = get_param(sys,'LastModifiedDate');
      | if isempty(last)
      |     last = datestr(now,'yyyy');
      | else
      |     last = last(end-3:end);
      | end
      | 
      | if strcmp(first,last)
      |     fprintf('%s -- Copyright %s Nexteer',NxtrConf,first)
      | else
      |     fprintf('%s -- %s%s- %s Nexteer',NxtrConf,char(169),first,last)
      | end
  Data Type Conversion : DataTypeConversion  OutDataTypeStr=uint8
  NoFlt : Constant  RequirementInfo={} %GIDa_9e7d5d77_5fe4_4375_b2fc_9d415667b1b0  Value=ELECGLBPRM_NOFLT_CNT_U08  OutDataTypeStr=uint8
  NoFlt2 : Constant  RequirementInfo={} %GIDa_ccecf245_c6d3_48bb_930a_2fb4228a5e26  Value=ELECGLBPRM_HWAGCENTROFFS_HWDEG_F32
  NtcSts : simulink/Sources/Enumerated Constant  OutDataTypeStr=Enum: NtcSts1  Value=NtcSts1.NTCSTS_PREPASSD  SampleTime=inf
  ShiftR : ArithShift  BitShiftNumber=1  BitShiftDirection=Right
  HwAg1Meas : Outport  OutDataTypeStr=single
  HwAg1TestOk : Outport  Port=2  OutDataTypeStr=uint8
  ParamByte : Outport  Port=3
  wires:
  Add/1 -> ShiftR/1
  ShiftR/1 -> Add1/1
  HwAg1Snsr0Abs/1 -> Add/1
  HwAg1Snsr1Abs/1 -> Add/2
  NoFlt/1 -> ParamByte/1
  NtcSts/1 -> Data Type Conversion/1
  Data Type Conversion/1 -> HwAg1TestOk/1
  NoFlt2/1 -> Add1/2
  Add1/1 -> HwAg1Meas/1

== system CM670A_HwAg1Meas/HwAg1Meas/HwAg1MeasPer4/HwAgRead/If Action Subsystem/AdjStepCalc/Diagc/If Action /finalAbsAg/If Action Subsystem1 ==
  Action Port : ActionPort  ActionType=else
  CopyRight2 : Subsystem  Description=|  mask(Copyright Information){none=on}
      | Copyright info block.                                               
      |                                                                     
      | Place copyright information at the top of every subsystem in design.
      mask prompts: none "No parameters"
      mask help: Place copyright information at the top of every subsystem in design.
      mask Display:
      | NxtrConf = 'Nexteer Confidential';
      | 
      | sys = bdroot; %handle for the current model ("system")
      | first = get_param(sys,'Created');
      | first = first(end-3:end);  %year is last four digits
      | 
      | last = get_param(sys,'LastModifiedDate');
      | if isempty(last)
      |     last = datestr(now,'yyyy');
      | else
      |     last = last(end-3:end);
      | end
      | 
      | if strcmp(first,last)
      |     fprintf('%s -- Copyright %s Nexteer',NxtrConf,first)
      | else
      |     fprintf('%s -- %s%s- %s Nexteer',NxtrConf,char(169),first,last)
      | end
  Data Type Conversion : DataTypeConversion  OutDataTypeStr=uint8
  Flt : Constant  Value=ELECGLBPRM_VRNRERRFLT_CNT_U08
  HwAg1 : Constant  Value=0  OutDataTypeStr=single
  NtcSts : simulink/Sources/Enumerated Constant  OutDataTypeStr=Enum: NtcSts1  Value=NtcSts1.NTCSTS_PREFAILD  SampleTime=inf
  HwAg1Meas : Outport
  HwAg1TestOk : Outport  Port=2  OutDataTypeStr=uint8
  ParamByte : Outport  Port=3  OutDataTypeStr=uint8
  wires:
  NtcSts/1 -> Data Type Conversion/1
  Flt/1 -> ParamByte/1
  HwAg1/1 -> HwAg1Meas/1
  Data Type Conversion/1 -> HwAg1TestOk/1

== system CM670A_HwAg1Meas/HwAg1Meas/HwAg1MeasPer4/HwAgRead/If Action Subsystem/AdjStepCalc/Diagc/If Action /finalAbsAg/If Action Subsystem/CopyRight2 ==

== system CM670A_HwAg1Meas/HwAg1Meas/HwAg1MeasPer4/HwAgRead/If Action Subsystem/AdjStepCalc/Diagc/If Action /finalAbsAg/If Action Subsystem1/CopyRight2 ==

== stateflow chart CM670A_HwAg1Meas/HwAg1Meas/HwAg1MeasPer2/Snsr0Read/SetNtcSts/ISO Fault Debounce Design ==
  settings: stateMachineType=MEALY_MACHINE
  note: NTCSTS_PASSD           (0)
      | NTCSTS_FAILD             (1)
      | NTCSTS_PREPASSD   (2)
      | NTCSTS_PREFAILD     (3)
      |
      | SIGQLFR_NORES        (0)
      | SIGQLFR_PASSD         (1)
      | SIGQLFR_FAILD           (2)
  note: Pass Loop
  note: Fail Loop
  note: 
  (default) -> (junction 89)
  (junction 89) -> (junction 95) [order 1] : [NtcSts ==3]
  (junction 89) -> (junction 93) [order 2] : [NtcSts ==2]
  (junction 89) -> (junction 141) [order 3] : [NtcSts ==1]
      | { ErrAcc = 32767;
      | Qualifier =2;
      |  }
  (junction 89) -> (junction 141) [order 4] : [NtcSts ==0]
      | { ErrAcc = -32768;
      | Qualifier=1;
      | }
  (junction 95) -> (junction 103) [order 2]
  (junction 95) -> (junction 111) [order 1] : [ErrAcc <=0]
      | {ErrAcc = DebStep;}
  (junction 93) -> (junction 123) [order 2] : {
      | ErrAcc = ErrAcc - DebStep;
      | }
  (junction 93) -> (junction 123) [order 1] : [(ErrAcc - DebStep) <= -32768]
      | { ErrAcc = -32768;
      | Qualifier=1;
      | }
  (junction 103) -> (junction 111) [order 1] : [(ErrAcc + DebStep) <32767]
      | {ErrAcc = ErrAcc + DebStep;}
  (junction 103) -> (junction 111) [order 2] : {ErrAcc = 32767;
      | Qualifier =2;}
  (junction 123) -> (junction 141)
  (junction 111) -> (junction 141)
  (junction 141) -> (junction 159) [order 2] : {ErrAcc = 0;
      | Qualifier =0;
      | }
  (junction 141) -> (junction 159) [order 1] : [SvcClr ==0]
  data: NtcSts input uint8; Qualifier output uint8; DebStep input uint16; ErrAcc local single; SvcClr input

== stateflow chart CM670A_HwAg1Meas/HwAg1Meas/HwAg1MeasPer3/Snsr1Read/SetNtcSts/ISO Fault Debounce Design ==
  settings: stateMachineType=MEALY_MACHINE
  note: NTCSTS_PASSD           (0)
      | NTCSTS_FAILD             (1)
      | NTCSTS_PREPASSD   (2)
      | NTCSTS_PREFAILD     (3)
      |
      | SIGQLFR_NORES        (0)
      | SIGQLFR_PASSD         (1)
      | SIGQLFR_FAILD           (2)
  note: Pass Loop
  note: Fail Loop
  note: 
  (default) -> (junction 89)
  (junction 89) -> (junction 95) [order 1] : [NtcSts ==3]
  (junction 89) -> (junction 93) [order 2] : [NtcSts ==2]
  (junction 89) -> (junction 141) [order 3] : [NtcSts ==1]
      | { ErrAcc = 32767;
      | Qualifier =2;
      |  }
  (junction 89) -> (junction 141) [order 4] : [NtcSts ==0]
      | { ErrAcc = -32768;
      | Qualifier=1;
      | }
  (junction 95) -> (junction 103) [order 2]
  (junction 95) -> (junction 111) [order 1] : [ErrAcc <=0]
      | {ErrAcc = DebStep;}
  (junction 93) -> (junction 123) [order 2] : {
      | ErrAcc = ErrAcc - DebStep;
      | }
  (junction 93) -> (junction 123) [order 1] : [(ErrAcc - DebStep) <= -32768]
      | { ErrAcc = -32768;
      | Qualifier=1;
      | }
  (junction 103) -> (junction 111) [order 1] : [(ErrAcc + DebStep) <32767]
      | {ErrAcc = ErrAcc + DebStep;}
  (junction 103) -> (junction 111) [order 2] : {ErrAcc = 32767;
      | Qualifier =2;}
  (junction 123) -> (junction 141)
  (junction 111) -> (junction 141)
  (junction 141) -> (junction 159) [order 2] : {ErrAcc = 0;
      | Qualifier =0;
      | }
  (junction 141) -> (junction 159) [order 1] : [SvcClr ==0]
  data: NtcSts input uint8; Qualifier output uint8; DebStep input uint16; ErrAcc local single; SvcClr input
